simulink model "sampleModel1562"  (R2023a)
settings: Solver=VariableStepAuto  StartTime=0.0  StopTime=10.0  RelTol=1e-3
libraries: hdlsllib x8, simulink x3
settings Model: Creator=user1  LastModifiedBy=user1

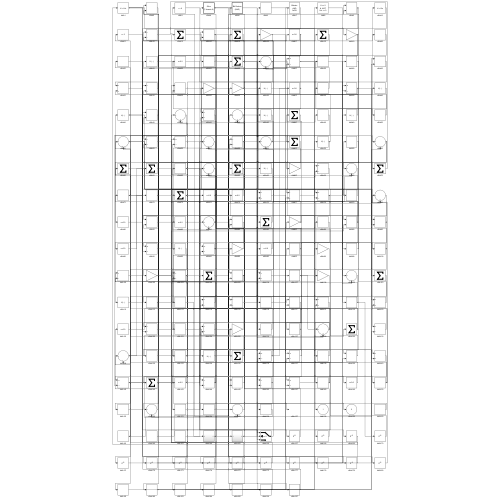
[thumbnail: Simulink's stored preview of the top-level diagram]
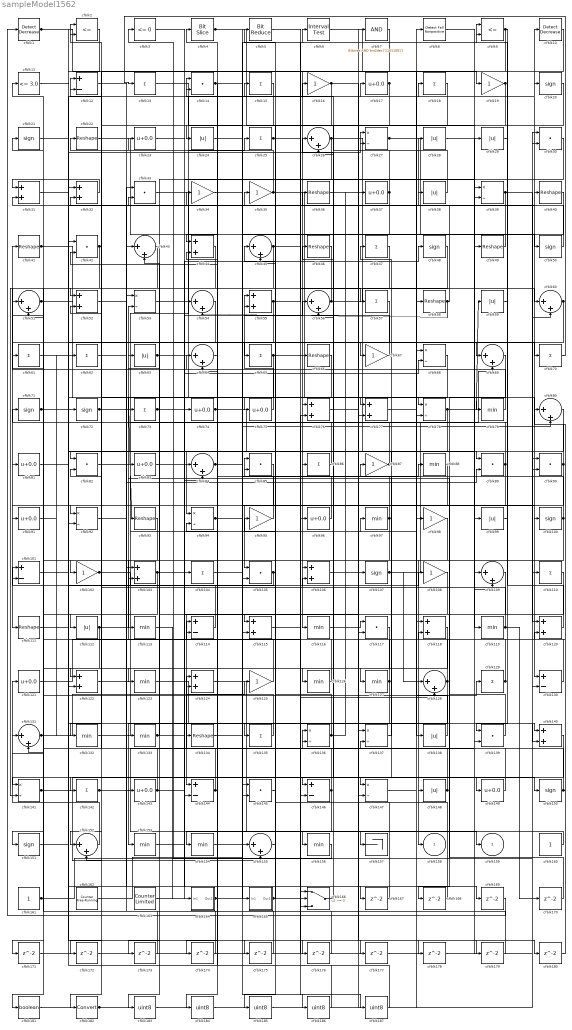
== system sampleModel1562 ==
  cfblk1 : simulink/Logic and Bit Operations/Detect Decrease  vinit=0.0  OutDataTypeStr=boolean
      settings: LibrarySourceBlock=|
      | hdlsllib/Logic and Bit
      | Operations/Detect
      | Decrease
  cfblk10 : simulink/Logic and Bit Operations/Detect Decrease  vinit=0.0  OutDataTypeStr=boolean
      settings: LibrarySourceBlock=|
      | hdlsllib/Logic and Bit
      | Operations/Detect
      | Decrease
  cfblk{20..21,48,50,71..72,100,107,150..151} (10 alike) : Signum
  cfblk{12,101,114,130,144,146} (6 alike) : Sum  Inputs=+-
  cfblk{16,19,34..35,67,87,95,98,102,108,125} (11 alike) : Gain
  cfblk{31..32,44,52,55,76..77,103,106,115,118,120,122,124,140} (15 alike) : Sum
  cfblk{13,15,18,25,47,57,61..62,65,70,73,86,104,110,129,135,142} (17 alike) : Sum  Inputs=+
  cfblk{14,30,33,42,82,85,89..90,105,117,139,145} (12 alike) : DotProduct  OutDataTypeStr=Inherit: Inherit via internal rule
  cfblk{26,43,45,51,54,56,60,64,69,80,84,109,128,131,152,155} (16 alike) : Sum  Inputs=|++
  cfblk11 : hdlsllib/Logic and Bit Operations/Compare To Constant  relop=<=  const=3.0  OutDataTypeStr=boolean
  cfblk{22,36,40..41,46,49,58,66,93,111,134} (11 alike) : Reshape
  cfblk{24,28..29,38,59,63,99,112,138,148} (10 alike) : Abs  SaturateOnIntegerOverflow=off
  cfblk{79,88,97,113,116,119,123,126..127,132..133,153..154,156} (14 alike) : MinMax
  cfblk{17,23,37,74..75,81,83,91,96,121,143,149} (12 alike) : Bias  Bias=0.0  SaturateOnIntegerOverflow=off
  cfblk{27,39,53,68,78,92,94,136..137,141,147} (11 alike) : Product  Inputs=*/  RndMeth=Zero  SaturateOnIntegerOverflow=on
  cfblk157 : Terminator
  cfblk160 : Constant  SampleTime=-1
  cfblk161 : Constant  SampleTime=-1
  cfblk162 : hdlsllib/Sources/Counter Free-Running  NumBits=16  tsamp=-1
  cfblk163 : hdlsllib/Sources/Counter Limited  uplimit=7  tsamp=-1
  cfblk164 : Subsystem
      settings: LibrarySourceBlock=|
      | hdlsllib/Ports &
      | Subsystems/Subsystem
  cfblk165 : Subsystem
      settings: LibrarySourceBlock=|
      | hdlsllib/Ports &
      | Subsystems/Subsystem
  cfblk166 : Switch  SaturateOnIntegerOverflow=off  InputSameDT=off
  cfblk{167..180} (14 alike) : Delay  SampleTime=1
  cfblk181 : DataTypeConversion  OutDataTypeStr=boolean  SaturateOnIntegerOverflow=off  RndMeth=Floor
  cfblk182 : DataTypeConversion  SaturateOnIntegerOverflow=off  RndMeth=Floor
  cfblk{183..187} (5 alike) : DataTypeConversion  OutDataTypeStr=uint8  SaturateOnIntegerOverflow=off  RndMeth=Floor
  cfblk2 : RelationalOperator  Operator=<=  OutDataTypeStr=boolean  InputSameDT=off
  cfblk3 : hdlsllib/Logic and Bit Operations/Compare To Zero  relop=<=  OutDataTypeStr=boolean
  cfblk4 : hdlsllib/Logic and Bit Operations/Bit Slice  lidx=7  ridx=0
  cfblk5 : hdlsllib/Logic and Bit Operations/Bit Reduce  mode=AND
  cfblk6 : hdlsllib/Logic and Bit Operations/Interval Test  IntervalClosedRight=on  uplimit=0.5  IntervalClosedLeft=on  lowlimit=-0.5  OutDataTypeStr=boolean
  cfblk7 : simulink/Logic and Bit Operations/Bitwise Operator  logicop=AND  UseBitMask=on  BitMask=bin2dec('11011001')  BitMaskRealWorld=Stored Integer
      settings: LibrarySourceBlock=|
      | hdlsllib/Logic and Bit
      | Operations/Bitwise
      | Operator
  cfblk8 : hdlsllib/Logic and Bit Operations/Detect Fall Nonpositive  vinit=0  OutDataTypeStr=boolean
  cfblk9 : RelationalOperator  Operator=<=  OutDataTypeStr=boolean  InputSameDT=off
  cfblk158 : Outport  VectorParamsAs1DForOutWhenUnconnected=off
  cfblk159 : Outport  Port=2  VectorParamsAs1DForOutWhenUnconnected=off
  wires:
  cfblk124/1 -> cfblk157/1
  cfblk113/1 -> cfblk164/1(In1)
  cfblk156/1 -> cfblk3/1
  cfblk90/1 -> cfblk10/1, cfblk127/1
  cfblk41/1 -> cfblk145/1, cfblk175/1
  cfblk163/1 -> cfblk74/1
  cfblk99/1 -> cfblk9/1
  cfblk91/1 -> cfblk72/1
  cfblk66/1 -> cfblk102/1
  cfblk98/1 -> cfblk158/1
  cfblk53/1 -> cfblk25/1
  cfblk101/1 -> cfblk140/1
  cfblk19/1 -> cfblk142/1, cfblk184/1
  cfblk28/1 -> cfblk99/1
  cfblk85/1 -> cfblk105/1
  cfblk109/1 -> cfblk144/1
  cfblk71/1 -> cfblk40/1, cfblk51/2, cfblk86/1
  cfblk10/1 -> cfblk116/1
  cfblk43/1 -> cfblk82/1
  cfblk83/1 -> cfblk94/1
  cfblk144/1 -> cfblk11/1, cfblk124/2
  cfblk79/1 -> cfblk41/1
  cfblk89/1 -> cfblk111/1, cfblk26/1, cfblk52/2
  cfblk130/1 -> cfblk53/2
  cfblk35/1 -> cfblk78/1, cfblk23/1
  cfblk142/1 -> cfblk159/1, cfblk49/1
  cfblk68/1 -> cfblk112/1
  cfblk118/1 -> cfblk148/1
  cfblk121/1 -> cfblk96/1
  cfblk112/1 -> cfblk20/1, cfblk171/1
  cfblk160/1 -> cfblk154/1
  cfblk72/1 -> cfblk93/1, cfblk152/2
  cfblk155/1 -> cfblk95/1
  cfblk78/1 -> cfblk59/1, cfblk147/1
  cfblk63/1 -> cfblk130/1, cfblk166/2
  cfblk22/1 -> cfblk50/1
  cfblk16/1 -> cfblk152/1, cfblk179/1
  cfblk15/1 -> cfblk24/1
  cfblk95/1 -> cfblk22/1
  cfblk97/1 -> cfblk4/1, cfblk147/2
  cfblk115/1 -> cfblk97/1
  cfblk33/1 -> cfblk165/1(In1)
  cfblk133/1 -> cfblk63/1, cfblk166/3
  cfblk153/1 -> cfblk48/1
  cfblk44/1 -> cfblk91/1
  cfblk138/1 -> cfblk21/1
  cfblk67/1 -> cfblk55/1
  cfblk137/1 -> cfblk87/1
  cfblk27/1 -> cfblk90/1, cfblk79/1
  cfblk122/1 -> cfblk8/1
  cfblk76/1 -> cfblk107/1
  cfblk146/1 -> cfblk156/1, cfblk14/2
  cfblk127/1 -> cfblk153/1, cfblk114/2
  cfblk61/1 -> cfblk120/1
  cfblk21/1 -> cfblk78/2
  cfblk40/1 -> cfblk76/1
  cfblk88/1 -> cfblk146/1
  cfblk8/1 -> cfblk119/1
  cfblk119/1 -> cfblk12/1, cfblk170/1
  cfblk129/1 -> cfblk82/2, cfblk43/2
  cfblk100/1 -> cfblk113/1, cfblk42/2
  cfblk161/1 -> cfblk51/1, cfblk60/2
  cfblk49/1 -> cfblk28/1
  cfblk152/1 -> cfblk121/1
  cfblk140/1 -> cfblk141/1
  cfblk128/1 -> cfblk144/2, cfblk103/2, cfblk126/1, cfblk123/1
  cfblk29/1 -> cfblk69/1
  cfblk42/1 -> cfblk12/2, cfblk131/2
  cfblk17/1 -> cfblk92/1, cfblk26/2
  cfblk141/1 -> cfblk149/1, cfblk155/2
  cfblk57/1 -> cfblk122/1
  cfblk143/1 -> cfblk32/2, cfblk68/2
  cfblk54/1 -> cfblk73/1
  cfblk3/1 -> cfblk39/2
  cfblk107/1 -> cfblk29/1, cfblk128/1
  cfblk116/1 -> cfblk117/1
  cfblk114/1 -> cfblk101/1
  cfblk87/1 -> cfblk46/1, cfblk47/1
  cfblk166/1 -> cfblk136/1
  cfblk51/1 -> cfblk166/1, cfblk84/2
  cfblk92/1 -> cfblk43/1
  cfblk93/1 -> cfblk151/1
  cfblk23/1 -> cfblk115/1
  cfblk25/1 -> cfblk128/2, cfblk187/1
  cfblk55/1 -> cfblk81/1, cfblk9/2
  cfblk149/1 -> cfblk124/1
  cfblk39/1 -> cfblk90/2, cfblk33/2
  cfblk6/1 -> cfblk19/1
  cfblk60/1 -> cfblk143/1, cfblk174/1
  cfblk52/1 -> cfblk150/1
  cfblk26/1 -> cfblk109/1, cfblk65/1
  cfblk73/1 -> cfblk56/1, cfblk117/2
  cfblk106/1 -> cfblk137/1
  cfblk62/1 -> cfblk77/1
  cfblk7/1 -> cfblk182/1
  cfblk126/1 -> cfblk64/1
  cfblk13/1 -> cfblk155/1
  cfblk45/1 -> cfblk134/1, cfblk57/1
  cfblk9/1 -> cfblk146/2, cfblk89/1
  cfblk37/1 -> cfblk16/1, cfblk145/2
  cfblk125/1 -> cfblk61/1
  cfblk162/1 -> cfblk18/1
  cfblk20/1 -> cfblk106/1
  cfblk77/1 -> cfblk58/1
  cfblk38/1 -> cfblk14/1
  cfblk120/1 -> cfblk71/1
  cfblk148/1 -> cfblk85/1, cfblk56/2
  cfblk80/1 -> cfblk122/2
  cfblk64/1 -> cfblk84/1
  cfblk131/1 -> cfblk125/1, cfblk62/1
  cfblk4/1 -> cfblk109/2, cfblk80/2
  cfblk81/1 -> cfblk17/1
  cfblk123/1 -> cfblk135/1
  cfblk65/1 -> cfblk132/1, cfblk140/2
  cfblk105/1 -> cfblk45/1, cfblk101/2
  cfblk75/1 -> cfblk55/2
  cfblk103/1 -> cfblk104/1, cfblk181/1
  cfblk132/1 -> cfblk54/1
  cfblk84/1 -> cfblk27/1, cfblk44/2
  cfblk94/1 -> cfblk64/2, cfblk178/1
  cfblk82/1 -> cfblk69/2
  cfblk139/1 -> cfblk83/1
  cfblk154/1 -> cfblk105/2
  cfblk110/1 -> cfblk133/1
  cfblk74/1 -> cfblk138/1, cfblk100/1
  cfblk32/1 -> cfblk31/1
  cfblk104/1 -> cfblk6/1
  cfblk36/1 -> cfblk110/1
  cfblk111/1 -> cfblk108/1
  cfblk164/1(Out1) -> cfblk88/1, cfblk114/1
  cfblk18/1 -> cfblk75/1
  cfblk96/1 -> cfblk31/2
  cfblk59/1 -> cfblk139/1
  cfblk165/1(Out1) -> cfblk137/2, cfblk5/1
  cfblk102/1 -> cfblk106/2, cfblk89/2
  cfblk145/1 -> cfblk15/1
  cfblk46/1 -> cfblk115/2
  cfblk70/1 -> cfblk13/1
  cfblk47/1 -> cfblk141/2
  cfblk134/1 -> cfblk36/1
  cfblk136/1 -> cfblk35/1, cfblk37/1
  cfblk150/1 -> cfblk136/2, cfblk80/1
  cfblk135/1 -> cfblk94/2
  cfblk86/1 -> cfblk2/1
  cfblk14/1 -> cfblk44/1, cfblk180/1
  cfblk147/1 -> cfblk129/1
  cfblk1/1 -> cfblk118/1, cfblk70/1, cfblk67/1
  cfblk58/1 -> cfblk54/2, cfblk38/1
  cfblk31/1 -> cfblk27/2
  cfblk50/1 -> cfblk2/2
  cfblk56/1 -> cfblk60/1, cfblk52/1
  cfblk2/1 -> cfblk92/2
  cfblk5/1 -> cfblk66/1
  cfblk12/1 -> cfblk167/1
  cfblk167/1 -> cfblk85/2
  cfblk69/1 -> cfblk168/1
  cfblk168/1 -> cfblk45/2
  cfblk11/1 -> cfblk169/1
  cfblk169/1 -> cfblk1/1
  cfblk170/1 -> cfblk118/2
  cfblk171/1 -> cfblk76/2
  cfblk117/1 -> cfblk172/1
  cfblk172/1 -> cfblk130/2
  cfblk108/1 -> cfblk173/1
  cfblk173/1 -> cfblk131/1
  cfblk174/1 -> cfblk103/1
  cfblk175/1 -> cfblk53/1
  cfblk24/1 -> cfblk176/1
  cfblk176/1 -> cfblk32/1
  cfblk151/1 -> cfblk177/1
  cfblk177/1 -> cfblk39/1
  cfblk178/1 -> cfblk139/2
  cfblk179/1 -> cfblk33/1
  cfblk180/1 -> cfblk120/2
  cfblk181/1 -> cfblk7/1
  cfblk182/1 -> cfblk77/2, cfblk98/1
  cfblk30/1 -> cfblk183/1
  cfblk183/1 -> cfblk68/1
  cfblk184/1 -> cfblk30/1
  cfblk48/1 -> cfblk185/1
  cfblk185/1 -> cfblk30/2
  cfblk34/1 -> cfblk186/1
  cfblk186/1 -> cfblk42/1
  cfblk187/1 -> cfblk34/1

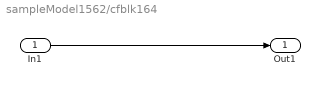
== system sampleModel1562/cfblk164 ==
  In1 : Inport
  Out1 : Outport
  wires:
  In1/1 -> Out1/1

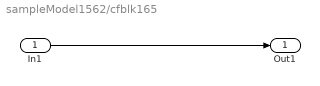
== system sampleModel1562/cfblk165 ==
  In1 : Inport
  Out1 : Outport
  wires:
  In1/1 -> Out1/1
